simulink model "tongbukongzhi2"  (R2014b)
settings: Solver=ode45  StartTime=0.0  StopTime=10.0  RelTol=1e-3
undefined symbols (not defined in the file): sigbuilder_block
libraries: simulink x89, fuzblock x41
(part 5 of 5)

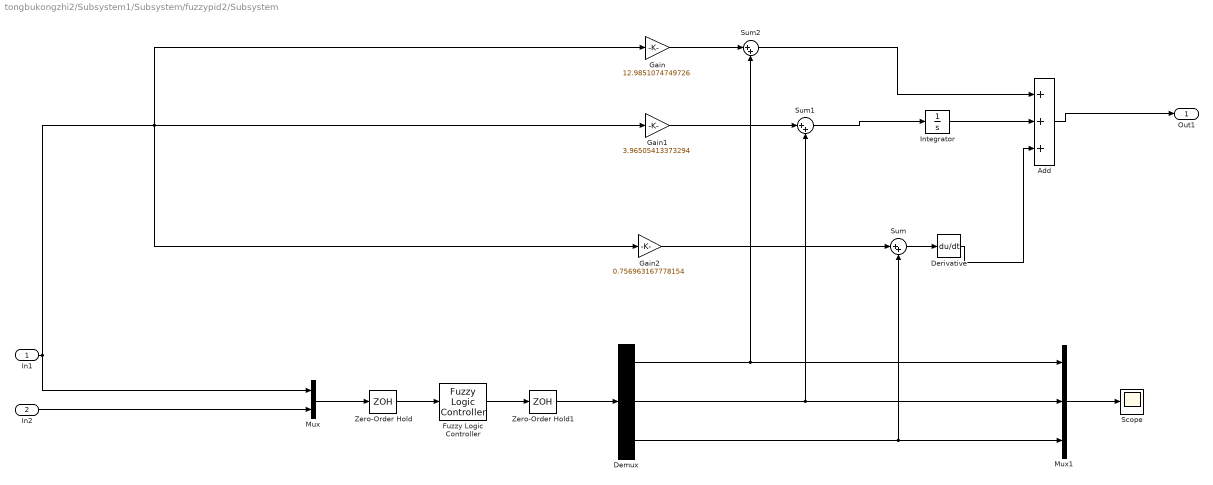
== system tongbukongzhi2/Subsystem1/Subsystem/fuzzypid2/Subsystem ==
  In1 : Inport
  In2 : Inport  Port=2
  Add : Sum  Inputs=+++
  Demux : Demux  Outputs=3
  Derivative : Derivative
  Fuzzy Logic Controller : fuzblock/Fuzzy Logic  Controller  fis=fuzzy1
  Gain : Gain  Gain=12.9851074749726
  Gain1 : Gain  Gain=3.96505413373294
  Gain2 : Gain  Gain=0.756963167778154
  Integrator : Integrator
  Mux : Mux  Inputs=2
  Mux1 : Mux  Inputs=3
  Scope : Scope
      settings: YMin=-0.2  YMax=0.05
  Sum : Sum  Inputs=|++
  Sum1 : Sum  Inputs=|++
  Sum2 : Sum  Inputs=|++
  Zero-Order Hold : ZeroOrderHold  SampleTime=0.1
  Zero-Order Hold1 : ZeroOrderHold  SampleTime=0.1
  Out1 : Outport
  wires:
  In1/1 -> Gain/1, Gain2/1, Gain1/1, Mux/1
  Derivative/1 -> Add/3
  Integrator/1 -> Add/2
  Add/1 -> Out1/1
  In2/1 -> Mux/2
  Gain/1 -> Sum2/1
  Sum2/1 -> Add/1
  Gain1/1 -> Sum1/1
  Sum1/1 -> Integrator/1
  Gain2/1 -> Sum/1
  Sum/1 -> Derivative/1
  Mux/1 -> Zero-Order Hold/1
  Fuzzy Logic Controller/1 -> Zero-Order Hold1/1
  Zero-Order Hold/1 -> Fuzzy Logic Controller/1
  Zero-Order Hold1/1 -> Demux/1
  Mux1/1 -> Scope/1
  Demux/3 -> Sum/2, Mux1/3
  Demux/2 -> Sum1/2, Mux1/2
  Demux/1 -> Mux1/1, Sum2/2

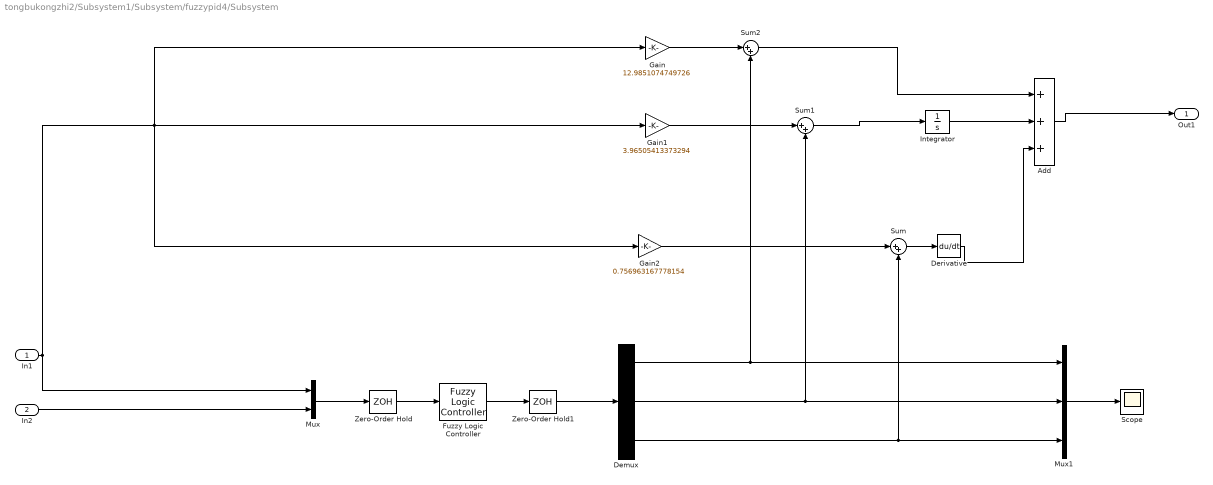
== system tongbukongzhi2/Subsystem1/Subsystem/fuzzypid4/Subsystem ==
  In1 : Inport
  In2 : Inport  Port=2
  Add : Sum  Inputs=+++
  Demux : Demux  Outputs=3
  Derivative : Derivative
  Fuzzy Logic Controller : fuzblock/Fuzzy Logic  Controller  fis=fuzzy1
  Gain : Gain  Gain=12.9851074749726
  Gain1 : Gain  Gain=3.96505413373294
  Gain2 : Gain  Gain=0.756963167778154
  Integrator : Integrator
  Mux : Mux  Inputs=2
  Mux1 : Mux  Inputs=3
  Scope : Scope
      settings: YMin=-0.2  YMax=0.05
  Sum : Sum  Inputs=|++
  Sum1 : Sum  Inputs=|++
  Sum2 : Sum  Inputs=|++
  Zero-Order Hold : ZeroOrderHold  SampleTime=0.1
  Zero-Order Hold1 : ZeroOrderHold  SampleTime=0.1
  Out1 : Outport
  wires:
  In1/1 -> Gain/1, Gain2/1, Gain1/1, Mux/1
  Derivative/1 -> Add/3
  Integrator/1 -> Add/2
  Add/1 -> Out1/1
  In2/1 -> Mux/2
  Gain/1 -> Sum2/1
  Sum2/1 -> Add/1
  Gain1/1 -> Sum1/1
  Sum1/1 -> Integrator/1
  Gain2/1 -> Sum/1
  Sum/1 -> Derivative/1
  Mux/1 -> Zero-Order Hold/1
  Fuzzy Logic Controller/1 -> Zero-Order Hold1/1
  Zero-Order Hold/1 -> Fuzzy Logic Controller/1
  Zero-Order Hold1/1 -> Demux/1
  Mux1/1 -> Scope/1
  Demux/3 -> Sum/2, Mux1/3
  Demux/2 -> Sum1/2, Mux1/2
  Demux/1 -> Mux1/1, Sum2/2

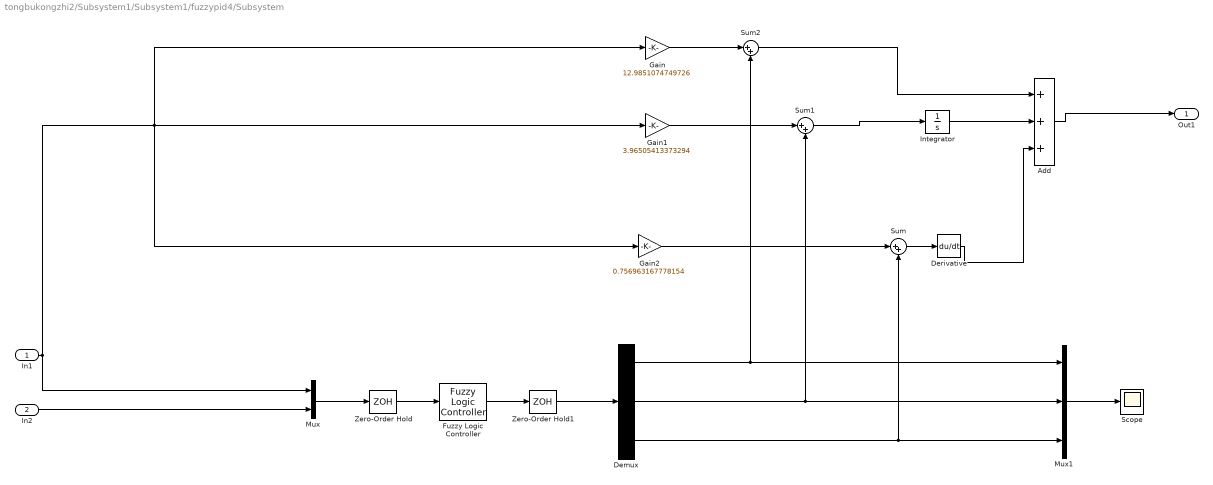
== system tongbukongzhi2/Subsystem1/Subsystem1/fuzzypid4/Subsystem ==
  In1 : Inport
  In2 : Inport  Port=2
  Add : Sum  Inputs=+++
  Demux : Demux  Outputs=3
  Derivative : Derivative
  Fuzzy Logic Controller : fuzblock/Fuzzy Logic  Controller  fis=fuzzy1
  Gain : Gain  Gain=12.9851074749726
  Gain1 : Gain  Gain=3.96505413373294
  Gain2 : Gain  Gain=0.756963167778154
  Integrator : Integrator
  Mux : Mux  Inputs=2
  Mux1 : Mux  Inputs=3
  Scope : Scope
      settings: YMin=-0.2  YMax=0.05
  Sum : Sum  Inputs=|++
  Sum1 : Sum  Inputs=|++
  Sum2 : Sum  Inputs=|++
  Zero-Order Hold : ZeroOrderHold  SampleTime=0.1
  Zero-Order Hold1 : ZeroOrderHold  SampleTime=0.1
  Out1 : Outport
  wires:
  In1/1 -> Gain/1, Gain2/1, Gain1/1, Mux/1
  Derivative/1 -> Add/3
  Integrator/1 -> Add/2
  Add/1 -> Out1/1
  In2/1 -> Mux/2
  Gain/1 -> Sum2/1
  Sum2/1 -> Add/1
  Gain1/1 -> Sum1/1
  Sum1/1 -> Integrator/1
  Gain2/1 -> Sum/1
  Sum/1 -> Derivative/1
  Mux/1 -> Zero-Order Hold/1
  Fuzzy Logic Controller/1 -> Zero-Order Hold1/1
  Zero-Order Hold/1 -> Fuzzy Logic Controller/1
  Zero-Order Hold1/1 -> Demux/1
  Mux1/1 -> Scope/1
  Demux/3 -> Sum/2, Mux1/3
  Demux/2 -> Sum1/2, Mux1/2
  Demux/1 -> Mux1/1, Sum2/2

== system tongbukongzhi2/Subsystem1/Subsystem1/fuzzypid5/Subsystem ==
  In1 : Inport
  In2 : Inport  Port=2
  Add : Sum  Inputs=+++
  Demux : Demux  Outputs=3
  Derivative : Derivative
  Fuzzy Logic Controller : fuzblock/Fuzzy Logic  Controller  fis=fuzzy1
  Gain : Gain  Gain=12.9851074749726
  Gain1 : Gain  Gain=3.96505413373294
  Gain2 : Gain  Gain=0.756963167778154
  Integrator : Integrator
  Mux : Mux  Inputs=2
  Mux1 : Mux  Inputs=3
  Scope : Scope
      settings: YMin=-0.2  YMax=0.05
  Sum : Sum  Inputs=|++
  Sum1 : Sum  Inputs=|++
  Sum2 : Sum  Inputs=|++
  Zero-Order Hold : ZeroOrderHold  SampleTime=0.1
  Zero-Order Hold1 : ZeroOrderHold  SampleTime=0.1
  Out1 : Outport
  wires:
  In1/1 -> Gain/1, Gain2/1, Gain1/1, Mux/1
  Derivative/1 -> Add/3
  Integrator/1 -> Add/2
  Add/1 -> Out1/1
  In2/1 -> Mux/2
  Gain/1 -> Sum2/1
  Sum2/1 -> Add/1
  Gain1/1 -> Sum1/1
  Sum1/1 -> Integrator/1
  Gain2/1 -> Sum/1
  Sum/1 -> Derivative/1
  Mux/1 -> Zero-Order Hold/1
  Fuzzy Logic Controller/1 -> Zero-Order Hold1/1
  Zero-Order Hold/1 -> Fuzzy Logic Controller/1
  Zero-Order Hold1/1 -> Demux/1
  Mux1/1 -> Scope/1
  Demux/3 -> Sum/2, Mux1/3
  Demux/2 -> Sum1/2, Mux1/2
  Demux/1 -> Mux1/1, Sum2/2

== system tongbukongzhi2/Subsystem1/Subsystem1/fuzzypid6/Subsystem ==
  In1 : Inport
  In2 : Inport  Port=2
  Add : Sum  Inputs=+++
  Demux : Demux  Outputs=3
  Derivative : Derivative
  Fuzzy Logic Controller : fuzblock/Fuzzy Logic  Controller  fis=fuzzy1
  Gain : Gain  Gain=12.9851074749726
  Gain1 : Gain  Gain=3.96505413373294
  Gain2 : Gain  Gain=0.756963167778154
  Integrator : Integrator
  Mux : Mux  Inputs=2
  Mux1 : Mux  Inputs=3
  Scope : Scope
      settings: YMin=-0.2  YMax=0.05
  Sum : Sum  Inputs=|++
  Sum1 : Sum  Inputs=|++
  Sum2 : Sum  Inputs=|++
  Zero-Order Hold : ZeroOrderHold  SampleTime=0.1
  Zero-Order Hold1 : ZeroOrderHold  SampleTime=0.1
  Out1 : Outport
  wires:
  In1/1 -> Gain/1, Gain2/1, Gain1/1, Mux/1
  Derivative/1 -> Add/3
  Integrator/1 -> Add/2
  Add/1 -> Out1/1
  In2/1 -> Mux/2
  Gain/1 -> Sum2/1
  Sum2/1 -> Add/1
  Gain1/1 -> Sum1/1
  Sum1/1 -> Integrator/1
  Gain2/1 -> Sum/1
  Sum/1 -> Derivative/1
  Mux/1 -> Zero-Order Hold/1
  Fuzzy Logic Controller/1 -> Zero-Order Hold1/1
  Zero-Order Hold/1 -> Fuzzy Logic Controller/1
  Zero-Order Hold1/1 -> Demux/1
  Mux1/1 -> Scope/1
  Demux/3 -> Sum/2, Mux1/3
  Demux/2 -> Sum1/2, Mux1/2
  Demux/1 -> Mux1/1, Sum2/2

== system tongbukongzhi2/Subsystem1/Subsystem12/fuzzypid1/Subsystem ==
  In1 : Inport
  In2 : Inport  Port=2
  Add : Sum  Inputs=+++
  Demux : Demux  Outputs=3
  Derivative : Derivative
  Fuzzy Logic Controller : fuzblock/Fuzzy Logic  Controller  fis=fuzzy1
  Gain : Gain  Gain=0.341898282831464
  Gain1 : Gain  Gain=4.22711463410027
  Gain2 : Gain  Gain=-0.0039506922991482
  Integrator : Integrator
  Mux : Mux  Inputs=2
  Mux1 : Mux  Inputs=3
  Scope : Scope
      settings: YMin=-0.2  YMax=0.05
  Sum : Sum  Inputs=|++
  Sum1 : Sum  Inputs=|++
  Sum2 : Sum  Inputs=|++
  Zero-Order Hold : ZeroOrderHold  SampleTime=0.1
  Zero-Order Hold1 : ZeroOrderHold  SampleTime=0.1
  Out1 : Outport
  wires:
  In1/1 -> Gain/1, Gain2/1, Gain1/1, Mux/1
  Derivative/1 -> Add/3
  Integrator/1 -> Add/2
  Add/1 -> Out1/1
  In2/1 -> Mux/2
  Gain/1 -> Sum2/1
  Sum2/1 -> Add/1
  Gain1/1 -> Sum1/1
  Sum1/1 -> Integrator/1
  Gain2/1 -> Sum/1
  Sum/1 -> Derivative/1
  Mux/1 -> Zero-Order Hold/1
  Fuzzy Logic Controller/1 -> Zero-Order Hold1/1
  Zero-Order Hold/1 -> Fuzzy Logic Controller/1
  Zero-Order Hold1/1 -> Demux/1
  Mux1/1 -> Scope/1
  Demux/3 -> Sum/2, Mux1/3
  Demux/2 -> Sum1/2, Mux1/2
  Demux/1 -> Mux1/1, Sum2/2

== system tongbukongzhi2/Subsystem1/Subsystem12/fuzzypid2/Subsystem ==
  In1 : Inport
  In2 : Inport  Port=2
  Add : Sum  Inputs=+++
  Demux : Demux  Outputs=3
  Derivative : Derivative
  Fuzzy Logic Controller : fuzblock/Fuzzy Logic  Controller  fis=fuzzy1
  Gain : Gain  Gain=0.341898282831464
  Gain1 : Gain  Gain=4.22711463410027
  Gain2 : Gain  Gain=-0.0039506922991482
  Integrator : Integrator
  Mux : Mux  Inputs=2
  Mux1 : Mux  Inputs=3
  Scope : Scope
      settings: YMin=-0.2  YMax=0.05
  Sum : Sum  Inputs=|++
  Sum1 : Sum  Inputs=|++
  Sum2 : Sum  Inputs=|++
  Zero-Order Hold : ZeroOrderHold  SampleTime=0.1
  Zero-Order Hold1 : ZeroOrderHold  SampleTime=0.1
  Out1 : Outport
  wires:
  In1/1 -> Gain/1, Gain2/1, Gain1/1, Mux/1
  Derivative/1 -> Add/3
  Integrator/1 -> Add/2
  Add/1 -> Out1/1
  In2/1 -> Mux/2
  Gain/1 -> Sum2/1
  Sum2/1 -> Add/1
  Gain1/1 -> Sum1/1
  Sum1/1 -> Integrator/1
  Gain2/1 -> Sum/1
  Sum/1 -> Derivative/1
  Mux/1 -> Zero-Order Hold/1
  Fuzzy Logic Controller/1 -> Zero-Order Hold1/1
  Zero-Order Hold/1 -> Fuzzy Logic Controller/1
  Zero-Order Hold1/1 -> Demux/1
  Mux1/1 -> Scope/1
  Demux/3 -> Sum/2, Mux1/3
  Demux/2 -> Sum1/2, Mux1/2
  Demux/1 -> Mux1/1, Sum2/2

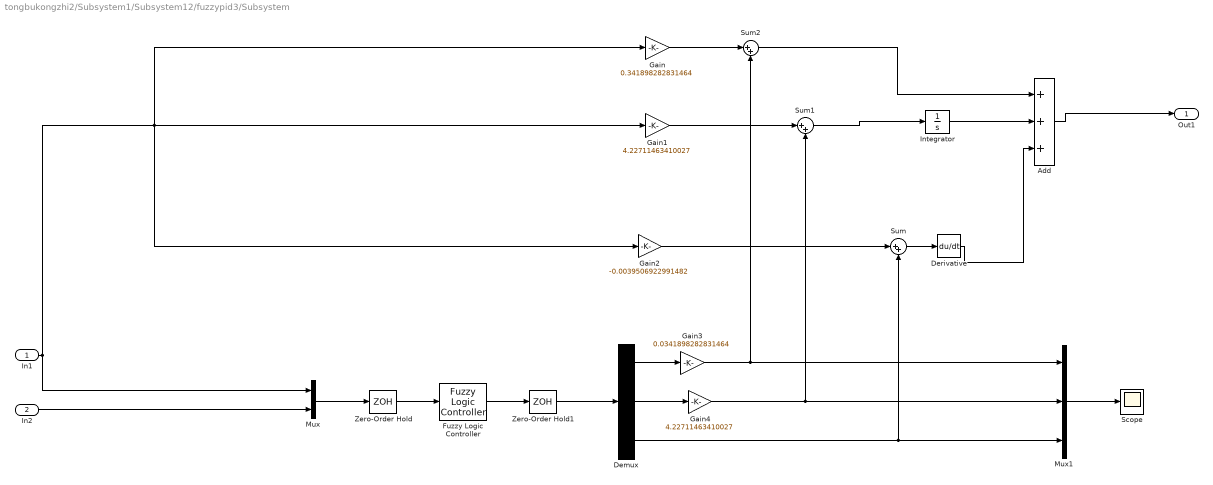
== system tongbukongzhi2/Subsystem1/Subsystem12/fuzzypid3/Subsystem ==
  In1 : Inport
  In2 : Inport  Port=2
  Add : Sum  Inputs=+++
  Demux : Demux  Outputs=3
  Derivative : Derivative
  Fuzzy Logic Controller : fuzblock/Fuzzy Logic  Controller  fis=fuzzy1
  Gain : Gain  Gain=0.341898282831464
  Gain1 : Gain  Gain=4.22711463410027
  Gain2 : Gain  Gain=-0.0039506922991482
  Gain3 : Gain  Gain=0.0341898282831464
  Gain4 : Gain  Gain=4.22711463410027
  Integrator : Integrator
  Mux : Mux  Inputs=2
  Mux1 : Mux  Inputs=3
  Scope : Scope
      settings: YMin=-0.2  YMax=0.05
  Sum : Sum  Inputs=|++
  Sum1 : Sum  Inputs=|++
  Sum2 : Sum  Inputs=|++
  Zero-Order Hold : ZeroOrderHold  SampleTime=0.1
  Zero-Order Hold1 : ZeroOrderHold  SampleTime=0.1
  Out1 : Outport
  wires:
  In1/1 -> Gain/1, Gain2/1, Gain1/1, Mux/1
  Derivative/1 -> Add/3
  Integrator/1 -> Add/2
  Add/1 -> Out1/1
  In2/1 -> Mux/2
  Gain/1 -> Sum2/1
  Sum2/1 -> Add/1
  Gain1/1 -> Sum1/1
  Sum1/1 -> Integrator/1
  Gain2/1 -> Sum/1
  Sum/1 -> Derivative/1
  Mux/1 -> Zero-Order Hold/1
  Fuzzy Logic Controller/1 -> Zero-Order Hold1/1
  Zero-Order Hold/1 -> Fuzzy Logic Controller/1
  Zero-Order Hold1/1 -> Demux/1
  Mux1/1 -> Scope/1
  Demux/3 -> Sum/2, Mux1/3
  Demux/2 -> Gain4/1
  Demux/1 -> Gain3/1
  Gain3/1 -> Mux1/1, Sum2/2
  Gain4/1 -> Sum1/2, Mux1/2

== system tongbukongzhi2/Subsystem1/Subsystem13/fuzzypid1/Subsystem ==
  In1 : Inport
  In2 : Inport  Port=2
  Add : Sum  Inputs=+++
  Demux : Demux  Outputs=3
  Derivative : Derivative
  Fuzzy Logic Controller : fuzblock/Fuzzy Logic  Controller  fis=fuzzy1
  Gain : Gain  Gain=0.341898282831464
  Gain1 : Gain  Gain=4.22711463410027
  Gain2 : Gain  Gain=-0.0039506922991482
  Integrator : Integrator
  Mux : Mux  Inputs=2
  Mux1 : Mux  Inputs=3
  Scope : Scope
      settings: YMin=-0.2  YMax=0.05
  Sum : Sum  Inputs=|++
  Sum1 : Sum  Inputs=|++
  Sum2 : Sum  Inputs=|++
  Zero-Order Hold : ZeroOrderHold  SampleTime=0.1
  Zero-Order Hold1 : ZeroOrderHold  SampleTime=0.1
  Out1 : Outport
  wires:
  In1/1 -> Gain/1, Gain2/1, Gain1/1, Mux/1
  Derivative/1 -> Add/3
  Integrator/1 -> Add/2
  Add/1 -> Out1/1
  In2/1 -> Mux/2
  Gain/1 -> Sum2/1
  Sum2/1 -> Add/1
  Gain1/1 -> Sum1/1
  Sum1/1 -> Integrator/1
  Gain2/1 -> Sum/1
  Sum/1 -> Derivative/1
  Mux/1 -> Zero-Order Hold/1
  Fuzzy Logic Controller/1 -> Zero-Order Hold1/1
  Zero-Order Hold/1 -> Fuzzy Logic Controller/1
  Zero-Order Hold1/1 -> Demux/1
  Mux1/1 -> Scope/1
  Demux/3 -> Sum/2, Mux1/3
  Demux/2 -> Sum1/2, Mux1/2
  Demux/1 -> Mux1/1, Sum2/2

== system tongbukongzhi2/Subsystem1/Subsystem13/fuzzypid2/Subsystem ==
  In1 : Inport
  In2 : Inport  Port=2
  Add : Sum  Inputs=+++
  Demux : Demux  Outputs=3
  Derivative : Derivative
  Fuzzy Logic Controller : fuzblock/Fuzzy Logic  Controller  fis=fuzzy1
  Gain : Gain  Gain=0.341898282831464
  Gain1 : Gain  Gain=4.22711463410027
  Gain2 : Gain  Gain=-0.0039506922991482
  Integrator : Integrator
  Mux : Mux  Inputs=2
  Mux1 : Mux  Inputs=3
  Scope : Scope
      settings: YMin=-0.2  YMax=0.05
  Sum : Sum  Inputs=|++
  Sum1 : Sum  Inputs=|++
  Sum2 : Sum  Inputs=|++
  Zero-Order Hold : ZeroOrderHold  SampleTime=0.1
  Zero-Order Hold1 : ZeroOrderHold  SampleTime=0.1
  Out1 : Outport
  wires:
  In1/1 -> Gain/1, Gain2/1, Gain1/1, Mux/1
  Derivative/1 -> Add/3
  Integrator/1 -> Add/2
  Add/1 -> Out1/1
  In2/1 -> Mux/2
  Gain/1 -> Sum2/1
  Sum2/1 -> Add/1
  Gain1/1 -> Sum1/1
  Sum1/1 -> Integrator/1
  Gain2/1 -> Sum/1
  Sum/1 -> Derivative/1
  Mux/1 -> Zero-Order Hold/1
  Fuzzy Logic Controller/1 -> Zero-Order Hold1/1
  Zero-Order Hold/1 -> Fuzzy Logic Controller/1
  Zero-Order Hold1/1 -> Demux/1
  Mux1/1 -> Scope/1
  Demux/3 -> Sum/2, Mux1/3
  Demux/2 -> Sum1/2, Mux1/2
  Demux/1 -> Mux1/1, Sum2/2

== system tongbukongzhi2/Subsystem1/Subsystem13/fuzzypid3/Subsystem ==
  In1 : Inport
  In2 : Inport  Port=2
  Add : Sum  Inputs=+++
  Demux : Demux  Outputs=3
  Derivative : Derivative
  Fuzzy Logic Controller : fuzblock/Fuzzy Logic  Controller  fis=fuzzy1
  Gain : Gain  Gain=0.341898282831464
  Gain1 : Gain  Gain=4.22711463410027
  Gain2 : Gain  Gain=-0.0039506922991482
  Integrator : Integrator
  Mux : Mux  Inputs=2
  Mux1 : Mux  Inputs=3
  Scope : Scope
      settings: YMin=-0.2  YMax=0.05
  Sum : Sum  Inputs=|++
  Sum1 : Sum  Inputs=|++
  Sum2 : Sum  Inputs=|++
  Zero-Order Hold : ZeroOrderHold  SampleTime=0.1
  Zero-Order Hold1 : ZeroOrderHold  SampleTime=0.1
  Out1 : Outport
  wires:
  In1/1 -> Gain/1, Gain2/1, Gain1/1, Mux/1
  Derivative/1 -> Add/3
  Integrator/1 -> Add/2
  Add/1 -> Out1/1
  In2/1 -> Mux/2
  Gain/1 -> Sum2/1
  Sum2/1 -> Add/1
  Gain1/1 -> Sum1/1
  Sum1/1 -> Integrator/1
  Gain2/1 -> Sum/1
  Sum/1 -> Derivative/1
  Mux/1 -> Zero-Order Hold/1
  Fuzzy Logic Controller/1 -> Zero-Order Hold1/1
  Zero-Order Hold/1 -> Fuzzy Logic Controller/1
  Zero-Order Hold1/1 -> Demux/1
  Mux1/1 -> Scope/1
  Demux/3 -> Sum/2, Mux1/3
  Demux/2 -> Sum1/2, Mux1/2
  Demux/1 -> Mux1/1, Sum2/2

== system tongbukongzhi2/Subsystem1/Subsystem14/fuzzypid1/Subsystem ==
  In1 : Inport
  In2 : Inport  Port=2
  Add : Sum  Inputs=+++
  Demux : Demux  Outputs=3
  Derivative : Derivative
  Fuzzy Logic Controller : fuzblock/Fuzzy Logic  Controller  fis=fuzzy1
  Gain : Gain  Gain=0.341898282831464
  Gain1 : Gain  Gain=4.22711463410027
  Gain2 : Gain  Gain=-0.0039506922991482
  Integrator : Integrator
  Mux : Mux  Inputs=2
  Mux1 : Mux  Inputs=3
  Scope : Scope
      settings: YMin=-0.2  YMax=0.05
  Sum : Sum  Inputs=|++
  Sum1 : Sum  Inputs=|++
  Sum2 : Sum  Inputs=|++
  Zero-Order Hold : ZeroOrderHold  SampleTime=0.1
  Zero-Order Hold1 : ZeroOrderHold  SampleTime=0.1
  Out1 : Outport
  wires:
  In1/1 -> Gain/1, Gain2/1, Gain1/1, Mux/1
  Derivative/1 -> Add/3
  Integrator/1 -> Add/2
  Add/1 -> Out1/1
  In2/1 -> Mux/2
  Gain/1 -> Sum2/1
  Sum2/1 -> Add/1
  Gain1/1 -> Sum1/1
  Sum1/1 -> Integrator/1
  Gain2/1 -> Sum/1
  Sum/1 -> Derivative/1
  Mux/1 -> Zero-Order Hold/1
  Fuzzy Logic Controller/1 -> Zero-Order Hold1/1
  Zero-Order Hold/1 -> Fuzzy Logic Controller/1
  Zero-Order Hold1/1 -> Demux/1
  Mux1/1 -> Scope/1
  Demux/3 -> Sum/2, Mux1/3
  Demux/2 -> Sum1/2, Mux1/2
  Demux/1 -> Mux1/1, Sum2/2

== system tongbukongzhi2/Subsystem1/Subsystem14/fuzzypid2/Subsystem ==
  In1 : Inport
  In2 : Inport  Port=2
  Add : Sum  Inputs=+++
  Demux : Demux  Outputs=3
  Derivative : Derivative
  Fuzzy Logic Controller : fuzblock/Fuzzy Logic  Controller  fis=fuzzy1
  Gain : Gain  Gain=0.341898282831464
  Gain1 : Gain  Gain=4.22711463410027
  Gain2 : Gain  Gain=-0.0039506922991482
  Integrator : Integrator
  Mux : Mux  Inputs=2
  Mux1 : Mux  Inputs=3
  Scope : Scope
      settings: YMin=-0.2  YMax=0.05
  Sum : Sum  Inputs=|++
  Sum1 : Sum  Inputs=|++
  Sum2 : Sum  Inputs=|++
  Zero-Order Hold : ZeroOrderHold  SampleTime=0.1
  Zero-Order Hold1 : ZeroOrderHold  SampleTime=0.1
  Out1 : Outport
  wires:
  In1/1 -> Gain/1, Gain2/1, Gain1/1, Mux/1
  Derivative/1 -> Add/3
  Integrator/1 -> Add/2
  Add/1 -> Out1/1
  In2/1 -> Mux/2
  Gain/1 -> Sum2/1
  Sum2/1 -> Add/1
  Gain1/1 -> Sum1/1
  Sum1/1 -> Integrator/1
  Gain2/1 -> Sum/1
  Sum/1 -> Derivative/1
  Mux/1 -> Zero-Order Hold/1
  Fuzzy Logic Controller/1 -> Zero-Order Hold1/1
  Zero-Order Hold/1 -> Fuzzy Logic Controller/1
  Zero-Order Hold1/1 -> Demux/1
  Mux1/1 -> Scope/1
  Demux/3 -> Sum/2, Mux1/3
  Demux/2 -> Sum1/2, Mux1/2
  Demux/1 -> Mux1/1, Sum2/2

== system tongbukongzhi2/Subsystem1/Subsystem14/fuzzypid3/Subsystem ==
  In1 : Inport
  In2 : Inport  Port=2
  Add : Sum  Inputs=+++
  Demux : Demux  Outputs=3
  Derivative : Derivative
  Fuzzy Logic Controller : fuzblock/Fuzzy Logic  Controller  fis=fuzzy1
  Gain : Gain  Gain=0.341898282831464
  Gain1 : Gain  Gain=4.22711463410027
  Gain2 : Gain  Gain=-0.0039506922991482
  Integrator : Integrator
  Mux : Mux  Inputs=2
  Mux1 : Mux  Inputs=3
  Scope : Scope
      settings: YMin=-0.2  YMax=0.05
  Sum : Sum  Inputs=|++
  Sum1 : Sum  Inputs=|++
  Sum2 : Sum  Inputs=|++
  Zero-Order Hold : ZeroOrderHold  SampleTime=0.1
  Zero-Order Hold1 : ZeroOrderHold  SampleTime=0.1
  Out1 : Outport
  wires:
  In1/1 -> Gain/1, Gain2/1, Gain1/1, Mux/1
  Derivative/1 -> Add/3
  Integrator/1 -> Add/2
  Add/1 -> Out1/1
  In2/1 -> Mux/2
  Gain/1 -> Sum2/1
  Sum2/1 -> Add/1
  Gain1/1 -> Sum1/1
  Sum1/1 -> Integrator/1
  Gain2/1 -> Sum/1
  Sum/1 -> Derivative/1
  Mux/1 -> Zero-Order Hold/1
  Fuzzy Logic Controller/1 -> Zero-Order Hold1/1
  Zero-Order Hold/1 -> Fuzzy Logic Controller/1
  Zero-Order Hold1/1 -> Demux/1
  Mux1/1 -> Scope/1
  Demux/3 -> Sum/2, Mux1/3
  Demux/2 -> Sum1/2, Mux1/2
  Demux/1 -> Mux1/1, Sum2/2

== system tongbukongzhi2/Subsystem1/Subsystem15/fuzzypid1/Subsystem ==
  In1 : Inport
  In2 : Inport  Port=2
  Add : Sum  Inputs=+++
  Demux : Demux  Outputs=3
  Derivative : Derivative
  Fuzzy Logic Controller : fuzblock/Fuzzy Logic  Controller  fis=fuzzy1
  Gain : Gain  Gain=0.341898282831464
  Gain1 : Gain  Gain=4.22711463410027
  Gain2 : Gain  Gain=-0.0039506922991482
  Integrator : Integrator
  Mux : Mux  Inputs=2
  Mux1 : Mux  Inputs=3
  Scope : Scope
      settings: YMin=-0.2  YMax=0.05
  Sum : Sum  Inputs=|++
  Sum1 : Sum  Inputs=|++
  Sum2 : Sum  Inputs=|++
  Zero-Order Hold : ZeroOrderHold  SampleTime=0.1
  Zero-Order Hold1 : ZeroOrderHold  SampleTime=0.1
  Out1 : Outport
  wires:
  In1/1 -> Gain/1, Gain2/1, Gain1/1, Mux/1
  Derivative/1 -> Add/3
  Integrator/1 -> Add/2
  Add/1 -> Out1/1
  In2/1 -> Mux/2
  Gain/1 -> Sum2/1
  Sum2/1 -> Add/1
  Gain1/1 -> Sum1/1
  Sum1/1 -> Integrator/1
  Gain2/1 -> Sum/1
  Sum/1 -> Derivative/1
  Mux/1 -> Zero-Order Hold/1
  Fuzzy Logic Controller/1 -> Zero-Order Hold1/1
  Zero-Order Hold/1 -> Fuzzy Logic Controller/1
  Zero-Order Hold1/1 -> Demux/1
  Mux1/1 -> Scope/1
  Demux/3 -> Sum/2, Mux1/3
  Demux/2 -> Sum1/2, Mux1/2
  Demux/1 -> Mux1/1, Sum2/2

== system tongbukongzhi2/Subsystem1/Subsystem15/fuzzypid2/Subsystem ==
  In1 : Inport
  In2 : Inport  Port=2
  Add : Sum  Inputs=+++
  Demux : Demux  Outputs=3
  Derivative : Derivative
  Fuzzy Logic Controller : fuzblock/Fuzzy Logic  Controller  fis=fuzzy1
  Gain : Gain  Gain=0.341898282831464
  Gain1 : Gain  Gain=4.22711463410027
  Gain2 : Gain  Gain=-0.0039506922991482
  Integrator : Integrator
  Mux : Mux  Inputs=2
  Mux1 : Mux  Inputs=3
  Scope : Scope
      settings: YMin=-0.2  YMax=0.05
  Sum : Sum  Inputs=|++
  Sum1 : Sum  Inputs=|++
  Sum2 : Sum  Inputs=|++
  Zero-Order Hold : ZeroOrderHold  SampleTime=0.1
  Zero-Order Hold1 : ZeroOrderHold  SampleTime=0.1
  Out1 : Outport
  wires:
  In1/1 -> Gain/1, Gain2/1, Gain1/1, Mux/1
  Derivative/1 -> Add/3
  Integrator/1 -> Add/2
  Add/1 -> Out1/1
  In2/1 -> Mux/2
  Gain/1 -> Sum2/1
  Sum2/1 -> Add/1
  Gain1/1 -> Sum1/1
  Sum1/1 -> Integrator/1
  Gain2/1 -> Sum/1
  Sum/1 -> Derivative/1
  Mux/1 -> Zero-Order Hold/1
  Fuzzy Logic Controller/1 -> Zero-Order Hold1/1
  Zero-Order Hold/1 -> Fuzzy Logic Controller/1
  Zero-Order Hold1/1 -> Demux/1
  Mux1/1 -> Scope/1
  Demux/3 -> Sum/2, Mux1/3
  Demux/2 -> Sum1/2, Mux1/2
  Demux/1 -> Mux1/1, Sum2/2

== system tongbukongzhi2/Subsystem1/Subsystem15/fuzzypid3/Subsystem ==
  In1 : Inport
  In2 : Inport  Port=2
  Add : Sum  Inputs=+++
  Demux : Demux  Outputs=3
  Derivative : Derivative
  Fuzzy Logic Controller : fuzblock/Fuzzy Logic  Controller  fis=fuzzy1
  Gain : Gain  Gain=0.341898282831464
  Gain1 : Gain  Gain=4.22711463410027
  Gain2 : Gain  Gain=-0.0039506922991482
  Integrator : Integrator
  Mux : Mux  Inputs=2
  Mux1 : Mux  Inputs=3
  Scope : Scope
      settings: YMin=-0.2  YMax=0.05
  Sum : Sum  Inputs=|++
  Sum1 : Sum  Inputs=|++
  Sum2 : Sum  Inputs=|++
  Zero-Order Hold : ZeroOrderHold  SampleTime=0.1
  Zero-Order Hold1 : ZeroOrderHold  SampleTime=0.1
  Out1 : Outport
  wires:
  In1/1 -> Gain/1, Gain2/1, Gain1/1, Mux/1
  Derivative/1 -> Add/3
  Integrator/1 -> Add/2
  Add/1 -> Out1/1
  In2/1 -> Mux/2
  Gain/1 -> Sum2/1
  Sum2/1 -> Add/1
  Gain1/1 -> Sum1/1
  Sum1/1 -> Integrator/1
  Gain2/1 -> Sum/1
  Sum/1 -> Derivative/1
  Mux/1 -> Zero-Order Hold/1
  Fuzzy Logic Controller/1 -> Zero-Order Hold1/1
  Zero-Order Hold/1 -> Fuzzy Logic Controller/1
  Zero-Order Hold1/1 -> Demux/1
  Mux1/1 -> Scope/1
  Demux/3 -> Sum/2, Mux1/3
  Demux/2 -> Sum1/2, Mux1/2
  Demux/1 -> Mux1/1, Sum2/2

== system tongbukongzhi2/Subsystem1/Subsystem16/fuzzypid1/Subsystem ==
  In1 : Inport
  In2 : Inport  Port=2
  Add : Sum  Inputs=+++
  Demux : Demux  Outputs=3
  Derivative : Derivative
  Fuzzy Logic Controller : fuzblock/Fuzzy Logic  Controller  fis=fuzzy1
  Gain : Gain  Gain=12.9851074749726
  Gain1 : Gain  Gain=3.96505413373294
  Gain2 : Gain  Gain=0.756963167778154
  Integrator : Integrator
  Mux : Mux  Inputs=2
  Mux1 : Mux  Inputs=3
  Scope : Scope
      settings: YMin=-0.2  YMax=0.05
  Sum : Sum  Inputs=|++
  Sum1 : Sum  Inputs=|++
  Sum2 : Sum  Inputs=|++
  Zero-Order Hold : ZeroOrderHold  SampleTime=0.1
  Zero-Order Hold1 : ZeroOrderHold  SampleTime=0.1
  Out1 : Outport
  wires:
  In1/1 -> Gain/1, Gain2/1, Gain1/1, Mux/1
  Derivative/1 -> Add/3
  Integrator/1 -> Add/2
  Add/1 -> Out1/1
  In2/1 -> Mux/2
  Gain/1 -> Sum2/1
  Sum2/1 -> Add/1
  Gain1/1 -> Sum1/1
  Sum1/1 -> Integrator/1
  Gain2/1 -> Sum/1
  Sum/1 -> Derivative/1
  Mux/1 -> Zero-Order Hold/1
  Fuzzy Logic Controller/1 -> Zero-Order Hold1/1
  Zero-Order Hold/1 -> Fuzzy Logic Controller/1
  Zero-Order Hold1/1 -> Demux/1
  Mux1/1 -> Scope/1
  Demux/3 -> Sum/2, Mux1/3
  Demux/2 -> Sum1/2, Mux1/2
  Demux/1 -> Mux1/1, Sum2/2

== system tongbukongzhi2/Subsystem1/Subsystem16/fuzzypid2/Subsystem ==
  In1 : Inport
  In2 : Inport  Port=2
  Add : Sum  Inputs=+++
  Demux : Demux  Outputs=3
  Derivative : Derivative
  Fuzzy Logic Controller : fuzblock/Fuzzy Logic  Controller  fis=fuzzy1
  Gain : Gain  Gain=12.9851074749726
  Gain1 : Gain  Gain=3.96505413373294
  Gain2 : Gain  Gain=0.756963167778154
  Integrator : Integrator
  Mux : Mux  Inputs=2
  Mux1 : Mux  Inputs=3
  Scope : Scope
      settings: YMin=-0.2  YMax=0.05
  Sum : Sum  Inputs=|++
  Sum1 : Sum  Inputs=|++
  Sum2 : Sum  Inputs=|++
  Zero-Order Hold : ZeroOrderHold  SampleTime=0.1
  Zero-Order Hold1 : ZeroOrderHold  SampleTime=0.1
  Out1 : Outport
  wires:
  In1/1 -> Gain/1, Gain2/1, Gain1/1, Mux/1
  Derivative/1 -> Add/3
  Integrator/1 -> Add/2
  Add/1 -> Out1/1
  In2/1 -> Mux/2
  Gain/1 -> Sum2/1
  Sum2/1 -> Add/1
  Gain1/1 -> Sum1/1
  Sum1/1 -> Integrator/1
  Gain2/1 -> Sum/1
  Sum/1 -> Derivative/1
  Mux/1 -> Zero-Order Hold/1
  Fuzzy Logic Controller/1 -> Zero-Order Hold1/1
  Zero-Order Hold/1 -> Fuzzy Logic Controller/1
  Zero-Order Hold1/1 -> Demux/1
  Mux1/1 -> Scope/1
  Demux/3 -> Sum/2, Mux1/3
  Demux/2 -> Sum1/2, Mux1/2
  Demux/1 -> Mux1/1, Sum2/2

== system tongbukongzhi2/Subsystem1/Subsystem16/fuzzypid4/Subsystem ==
  In1 : Inport
  In2 : Inport  Port=2
  Add : Sum  Inputs=+++
  Demux : Demux  Outputs=3
  Derivative : Derivative
  Fuzzy Logic Controller : fuzblock/Fuzzy Logic  Controller  fis=fuzzy1
  Gain : Gain  Gain=12.9851074749726
  Gain1 : Gain  Gain=3.96505413373294
  Gain2 : Gain  Gain=0.756963167778154
  Integrator : Integrator
  Mux : Mux  Inputs=2
  Mux1 : Mux  Inputs=3
  Scope : Scope
      settings: YMin=-0.2  YMax=0.05
  Sum : Sum  Inputs=|++
  Sum1 : Sum  Inputs=|++
  Sum2 : Sum  Inputs=|++
  Zero-Order Hold : ZeroOrderHold  SampleTime=0.1
  Zero-Order Hold1 : ZeroOrderHold  SampleTime=0.1
  Out1 : Outport
  wires:
  In1/1 -> Gain/1, Gain2/1, Gain1/1, Mux/1
  Derivative/1 -> Add/3
  Integrator/1 -> Add/2
  Add/1 -> Out1/1
  In2/1 -> Mux/2
  Gain/1 -> Sum2/1
  Sum2/1 -> Add/1
  Gain1/1 -> Sum1/1
  Sum1/1 -> Integrator/1
  Gain2/1 -> Sum/1
  Sum/1 -> Derivative/1
  Mux/1 -> Zero-Order Hold/1
  Fuzzy Logic Controller/1 -> Zero-Order Hold1/1
  Zero-Order Hold/1 -> Fuzzy Logic Controller/1
  Zero-Order Hold1/1 -> Demux/1
  Mux1/1 -> Scope/1
  Demux/3 -> Sum/2, Mux1/3
  Demux/2 -> Sum1/2, Mux1/2
  Demux/1 -> Mux1/1, Sum2/2

== system tongbukongzhi2/Subsystem1/Subsystem17/fuzzypid4/Subsystem ==
  In1 : Inport
  In2 : Inport  Port=2
  Add : Sum  Inputs=+++
  Demux : Demux  Outputs=3
  Derivative : Derivative
  Fuzzy Logic Controller : fuzblock/Fuzzy Logic  Controller  fis=fuzzy1
  Gain : Gain  Gain=12.9851074749726
  Gain1 : Gain  Gain=3.96505413373294
  Gain2 : Gain  Gain=0.756963167778154
  Integrator : Integrator
  Mux : Mux  Inputs=2
  Mux1 : Mux  Inputs=3
  Scope : Scope
      settings: YMin=-0.2  YMax=0.05
  Sum : Sum  Inputs=|++
  Sum1 : Sum  Inputs=|++
  Sum2 : Sum  Inputs=|++
  Zero-Order Hold : ZeroOrderHold  SampleTime=0.1
  Zero-Order Hold1 : ZeroOrderHold  SampleTime=0.1
  Out1 : Outport
  wires:
  In1/1 -> Gain/1, Gain2/1, Gain1/1, Mux/1
  Derivative/1 -> Add/3
  Integrator/1 -> Add/2
  Add/1 -> Out1/1
  In2/1 -> Mux/2
  Gain/1 -> Sum2/1
  Sum2/1 -> Add/1
  Gain1/1 -> Sum1/1
  Sum1/1 -> Integrator/1
  Gain2/1 -> Sum/1
  Sum/1 -> Derivative/1
  Mux/1 -> Zero-Order Hold/1
  Fuzzy Logic Controller/1 -> Zero-Order Hold1/1
  Zero-Order Hold/1 -> Fuzzy Logic Controller/1
  Zero-Order Hold1/1 -> Demux/1
  Mux1/1 -> Scope/1
  Demux/3 -> Sum/2, Mux1/3
  Demux/2 -> Sum1/2, Mux1/2
  Demux/1 -> Mux1/1, Sum2/2

== system tongbukongzhi2/Subsystem1/Subsystem17/fuzzypid5/Subsystem ==
  In1 : Inport
  In2 : Inport  Port=2
  Add : Sum  Inputs=+++
  Demux : Demux  Outputs=3
  Derivative : Derivative
  Fuzzy Logic Controller : fuzblock/Fuzzy Logic  Controller  fis=fuzzy1
  Gain : Gain  Gain=12.9851074749726
  Gain1 : Gain  Gain=3.96505413373294
  Gain2 : Gain  Gain=0.756963167778154
  Integrator : Integrator
  Mux : Mux  Inputs=2
  Mux1 : Mux  Inputs=3
  Scope : Scope
      settings: YMin=-0.2  YMax=0.05
  Sum : Sum  Inputs=|++
  Sum1 : Sum  Inputs=|++
  Sum2 : Sum  Inputs=|++
  Zero-Order Hold : ZeroOrderHold  SampleTime=0.1
  Zero-Order Hold1 : ZeroOrderHold  SampleTime=0.1
  Out1 : Outport
  wires:
  In1/1 -> Gain/1, Gain2/1, Gain1/1, Mux/1
  Derivative/1 -> Add/3
  Integrator/1 -> Add/2
  Add/1 -> Out1/1
  In2/1 -> Mux/2
  Gain/1 -> Sum2/1
  Sum2/1 -> Add/1
  Gain1/1 -> Sum1/1
  Sum1/1 -> Integrator/1
  Gain2/1 -> Sum/1
  Sum/1 -> Derivative/1
  Mux/1 -> Zero-Order Hold/1
  Fuzzy Logic Controller/1 -> Zero-Order Hold1/1
  Zero-Order Hold/1 -> Fuzzy Logic Controller/1
  Zero-Order Hold1/1 -> Demux/1
  Mux1/1 -> Scope/1
  Demux/3 -> Sum/2, Mux1/3
  Demux/2 -> Sum1/2, Mux1/2
  Demux/1 -> Mux1/1, Sum2/2

== system tongbukongzhi2/Subsystem1/Subsystem17/fuzzypid6/Subsystem ==
  In1 : Inport
  In2 : Inport  Port=2
  Add : Sum  Inputs=+++
  Demux : Demux  Outputs=3
  Derivative : Derivative
  Fuzzy Logic Controller : fuzblock/Fuzzy Logic  Controller  fis=fuzzy1
  Gain : Gain  Gain=12.9851074749726
  Gain1 : Gain  Gain=3.96505413373294
  Gain2 : Gain  Gain=0.756963167778154
  Integrator : Integrator
  Mux : Mux  Inputs=2
  Mux1 : Mux  Inputs=3
  Scope : Scope
      settings: YMin=-0.2  YMax=0.05
  Sum : Sum  Inputs=|++
  Sum1 : Sum  Inputs=|++
  Sum2 : Sum  Inputs=|++
  Zero-Order Hold : ZeroOrderHold  SampleTime=0.1
  Zero-Order Hold1 : ZeroOrderHold  SampleTime=0.1
  Out1 : Outport
  wires:
  In1/1 -> Gain/1, Gain2/1, Gain1/1, Mux/1
  Derivative/1 -> Add/3
  Integrator/1 -> Add/2
  Add/1 -> Out1/1
  In2/1 -> Mux/2
  Gain/1 -> Sum2/1
  Sum2/1 -> Add/1
  Gain1/1 -> Sum1/1
  Sum1/1 -> Integrator/1
  Gain2/1 -> Sum/1
  Sum/1 -> Derivative/1
  Mux/1 -> Zero-Order Hold/1
  Fuzzy Logic Controller/1 -> Zero-Order Hold1/1
  Zero-Order Hold/1 -> Fuzzy Logic Controller/1
  Zero-Order Hold1/1 -> Demux/1
  Mux1/1 -> Scope/1
  Demux/3 -> Sum/2, Mux1/3
  Demux/2 -> Sum1/2, Mux1/2
  Demux/1 -> Mux1/1, Sum2/2

== system tongbukongzhi2/Subsystem1/Subsystem18/fuzzypid4/Subsystem ==
  In1 : Inport
  In2 : Inport  Port=2
  Add : Sum  Inputs=+++
  Demux : Demux  Outputs=3
  Derivative : Derivative
  Fuzzy Logic Controller : fuzblock/Fuzzy Logic  Controller  fis=fuzzy1
  Gain : Gain  Gain=12.9851074749726
  Gain1 : Gain  Gain=3.96505413373294
  Gain2 : Gain  Gain=0.756963167778154
  Integrator : Integrator
  Mux : Mux  Inputs=2
  Mux1 : Mux  Inputs=3
  Scope : Scope
      settings: YMin=-0.2  YMax=0.05
  Sum : Sum  Inputs=|++
  Sum1 : Sum  Inputs=|++
  Sum2 : Sum  Inputs=|++
  Zero-Order Hold : ZeroOrderHold  SampleTime=0.1
  Zero-Order Hold1 : ZeroOrderHold  SampleTime=0.1
  Out1 : Outport
  wires:
  In1/1 -> Gain/1, Gain2/1, Gain1/1, Mux/1
  Derivative/1 -> Add/3
  Integrator/1 -> Add/2
  Add/1 -> Out1/1
  In2/1 -> Mux/2
  Gain/1 -> Sum2/1
  Sum2/1 -> Add/1
  Gain1/1 -> Sum1/1
  Sum1/1 -> Integrator/1
  Gain2/1 -> Sum/1
  Sum/1 -> Derivative/1
  Mux/1 -> Zero-Order Hold/1
  Fuzzy Logic Controller/1 -> Zero-Order Hold1/1
  Zero-Order Hold/1 -> Fuzzy Logic Controller/1
  Zero-Order Hold1/1 -> Demux/1
  Mux1/1 -> Scope/1
  Demux/3 -> Sum/2, Mux1/3
  Demux/2 -> Sum1/2, Mux1/2
  Demux/1 -> Mux1/1, Sum2/2

== system tongbukongzhi2/Subsystem1/Subsystem18/fuzzypid5/Subsystem ==
  In1 : Inport
  In2 : Inport  Port=2
  Add : Sum  Inputs=+++
  Demux : Demux  Outputs=3
  Derivative : Derivative
  Fuzzy Logic Controller : fuzblock/Fuzzy Logic  Controller  fis=fuzzy1
  Gain : Gain  Gain=12.9851074749726
  Gain1 : Gain  Gain=3.96505413373294
  Gain2 : Gain  Gain=0.756963167778154
  Integrator : Integrator
  Mux : Mux  Inputs=2
  Mux1 : Mux  Inputs=3
  Scope : Scope
      settings: YMin=-0.2  YMax=0.05
  Sum : Sum  Inputs=|++
  Sum1 : Sum  Inputs=|++
  Sum2 : Sum  Inputs=|++
  Zero-Order Hold : ZeroOrderHold  SampleTime=0.1
  Zero-Order Hold1 : ZeroOrderHold  SampleTime=0.1
  Out1 : Outport
  wires:
  In1/1 -> Gain/1, Gain2/1, Gain1/1, Mux/1
  Derivative/1 -> Add/3
  Integrator/1 -> Add/2
  Add/1 -> Out1/1
  In2/1 -> Mux/2
  Gain/1 -> Sum2/1
  Sum2/1 -> Add/1
  Gain1/1 -> Sum1/1
  Sum1/1 -> Integrator/1
  Gain2/1 -> Sum/1
  Sum/1 -> Derivative/1
  Mux/1 -> Zero-Order Hold/1
  Fuzzy Logic Controller/1 -> Zero-Order Hold1/1
  Zero-Order Hold/1 -> Fuzzy Logic Controller/1
  Zero-Order Hold1/1 -> Demux/1
  Mux1/1 -> Scope/1
  Demux/3 -> Sum/2, Mux1/3
  Demux/2 -> Sum1/2, Mux1/2
  Demux/1 -> Mux1/1, Sum2/2

== system tongbukongzhi2/Subsystem1/Subsystem18/fuzzypid6/Subsystem ==
  In1 : Inport
  In2 : Inport  Port=2
  Add : Sum  Inputs=+++
  Demux : Demux  Outputs=3
  Derivative : Derivative
  Fuzzy Logic Controller : fuzblock/Fuzzy Logic  Controller  fis=fuzzy1
  Gain : Gain  Gain=12.9851074749726
  Gain1 : Gain  Gain=3.96505413373294
  Gain2 : Gain  Gain=0.756963167778154
  Integrator : Integrator
  Mux : Mux  Inputs=2
  Mux1 : Mux  Inputs=3
  Scope : Scope
      settings: YMin=-0.2  YMax=0.05
  Sum : Sum  Inputs=|++
  Sum1 : Sum  Inputs=|++
  Sum2 : Sum  Inputs=|++
  Zero-Order Hold : ZeroOrderHold  SampleTime=0.1
  Zero-Order Hold1 : ZeroOrderHold  SampleTime=0.1
  Out1 : Outport
  wires:
  In1/1 -> Gain/1, Gain2/1, Gain1/1, Mux/1
  Derivative/1 -> Add/3
  Integrator/1 -> Add/2
  Add/1 -> Out1/1
  In2/1 -> Mux/2
  Gain/1 -> Sum2/1
  Sum2/1 -> Add/1
  Gain1/1 -> Sum1/1
  Sum1/1 -> Integrator/1
  Gain2/1 -> Sum/1
  Sum/1 -> Derivative/1
  Mux/1 -> Zero-Order Hold/1
  Fuzzy Logic Controller/1 -> Zero-Order Hold1/1
  Zero-Order Hold/1 -> Fuzzy Logic Controller/1
  Zero-Order Hold1/1 -> Demux/1
  Mux1/1 -> Scope/1
  Demux/3 -> Sum/2, Mux1/3
  Demux/2 -> Sum1/2, Mux1/2
  Demux/1 -> Mux1/1, Sum2/2

== system tongbukongzhi2/Subsystem1/Subsystem19/fuzzypid4/Subsystem ==
  In1 : Inport
  In2 : Inport  Port=2
  Add : Sum  Inputs=+++
  Demux : Demux  Outputs=3
  Derivative : Derivative
  Fuzzy Logic Controller : fuzblock/Fuzzy Logic  Controller  fis=fuzzy1
  Gain : Gain  Gain=12.9851074749726
  Gain1 : Gain  Gain=3.96505413373294
  Gain2 : Gain  Gain=0.756963167778154
  Integrator : Integrator
  Mux : Mux  Inputs=2
  Mux1 : Mux  Inputs=3
  Scope : Scope
      settings: YMin=-0.2  YMax=0.05
  Sum : Sum  Inputs=|++
  Sum1 : Sum  Inputs=|++
  Sum2 : Sum  Inputs=|++
  Zero-Order Hold : ZeroOrderHold  SampleTime=0.1
  Zero-Order Hold1 : ZeroOrderHold  SampleTime=0.1
  Out1 : Outport
  wires:
  In1/1 -> Gain/1, Gain2/1, Gain1/1, Mux/1
  Derivative/1 -> Add/3
  Integrator/1 -> Add/2
  Add/1 -> Out1/1
  In2/1 -> Mux/2
  Gain/1 -> Sum2/1
  Sum2/1 -> Add/1
  Gain1/1 -> Sum1/1
  Sum1/1 -> Integrator/1
  Gain2/1 -> Sum/1
  Sum/1 -> Derivative/1
  Mux/1 -> Zero-Order Hold/1
  Fuzzy Logic Controller/1 -> Zero-Order Hold1/1
  Zero-Order Hold/1 -> Fuzzy Logic Controller/1
  Zero-Order Hold1/1 -> Demux/1
  Mux1/1 -> Scope/1
  Demux/3 -> Sum/2, Mux1/3
  Demux/2 -> Sum1/2, Mux1/2
  Demux/1 -> Mux1/1, Sum2/2

== system tongbukongzhi2/Subsystem1/Subsystem19/fuzzypid5/Subsystem ==
  In1 : Inport
  In2 : Inport  Port=2
  Add : Sum  Inputs=+++
  Demux : Demux  Outputs=3
  Derivative : Derivative
  Fuzzy Logic Controller : fuzblock/Fuzzy Logic  Controller  fis=fuzzy1
  Gain : Gain  Gain=12.9851074749726
  Gain1 : Gain  Gain=3.96505413373294
  Gain2 : Gain  Gain=0.756963167778154
  Integrator : Integrator
  Mux : Mux  Inputs=2
  Mux1 : Mux  Inputs=3
  Scope : Scope
      settings: YMin=-0.2  YMax=0.05
  Sum : Sum  Inputs=|++
  Sum1 : Sum  Inputs=|++
  Sum2 : Sum  Inputs=|++
  Zero-Order Hold : ZeroOrderHold  SampleTime=0.1
  Zero-Order Hold1 : ZeroOrderHold  SampleTime=0.1
  Out1 : Outport
  wires:
  In1/1 -> Gain/1, Gain2/1, Gain1/1, Mux/1
  Derivative/1 -> Add/3
  Integrator/1 -> Add/2
  Add/1 -> Out1/1
  In2/1 -> Mux/2
  Gain/1 -> Sum2/1
  Sum2/1 -> Add/1
  Gain1/1 -> Sum1/1
  Sum1/1 -> Integrator/1
  Gain2/1 -> Sum/1
  Sum/1 -> Derivative/1
  Mux/1 -> Zero-Order Hold/1
  Fuzzy Logic Controller/1 -> Zero-Order Hold1/1
  Zero-Order Hold/1 -> Fuzzy Logic Controller/1
  Zero-Order Hold1/1 -> Demux/1
  Mux1/1 -> Scope/1
  Demux/3 -> Sum/2, Mux1/3
  Demux/2 -> Sum1/2, Mux1/2
  Demux/1 -> Mux1/1, Sum2/2

== system tongbukongzhi2/Subsystem1/Subsystem19/fuzzypid6/Subsystem ==
  In1 : Inport
  In2 : Inport  Port=2
  Add : Sum  Inputs=+++
  Demux : Demux  Outputs=3
  Derivative : Derivative
  Fuzzy Logic Controller : fuzblock/Fuzzy Logic  Controller  fis=fuzzy1
  Gain : Gain  Gain=12.9851074749726
  Gain1 : Gain  Gain=3.96505413373294
  Gain2 : Gain  Gain=0.756963167778154
  Integrator : Integrator
  Mux : Mux  Inputs=2
  Mux1 : Mux  Inputs=3
  Scope : Scope
      settings: YMin=-0.2  YMax=0.05
  Sum : Sum  Inputs=|++
  Sum1 : Sum  Inputs=|++
  Sum2 : Sum  Inputs=|++
  Zero-Order Hold : ZeroOrderHold  SampleTime=0.1
  Zero-Order Hold1 : ZeroOrderHold  SampleTime=0.1
  Out1 : Outport
  wires:
  In1/1 -> Gain/1, Gain2/1, Gain1/1, Mux/1
  Derivative/1 -> Add/3
  Integrator/1 -> Add/2
  Add/1 -> Out1/1
  In2/1 -> Mux/2
  Gain/1 -> Sum2/1
  Sum2/1 -> Add/1
  Gain1/1 -> Sum1/1
  Sum1/1 -> Integrator/1
  Gain2/1 -> Sum/1
  Sum/1 -> Derivative/1
  Mux/1 -> Zero-Order Hold/1
  Fuzzy Logic Controller/1 -> Zero-Order Hold1/1
  Zero-Order Hold/1 -> Fuzzy Logic Controller/1
  Zero-Order Hold1/1 -> Demux/1
  Mux1/1 -> Scope/1
  Demux/3 -> Sum/2, Mux1/3
  Demux/2 -> Sum1/2, Mux1/2
  Demux/1 -> Mux1/1, Sum2/2

== system tongbukongzhi2/Subsystem1/Subsystem2/fuzzypid4/Subsystem ==
  In1 : Inport
  In2 : Inport  Port=2
  Add : Sum  Inputs=+++
  Demux : Demux  Outputs=3
  Derivative : Derivative
  Fuzzy Logic Controller : fuzblock/Fuzzy Logic  Controller  fis=fuzzy1
  Gain : Gain  Gain=12.9851074749726
  Gain1 : Gain  Gain=3.96505413373294
  Gain2 : Gain  Gain=0.756963167778154
  Integrator : Integrator
  Mux : Mux  Inputs=2
  Mux1 : Mux  Inputs=3
  Scope : Scope
      settings: YMin=-0.2  YMax=0.05
  Sum : Sum  Inputs=|++
  Sum1 : Sum  Inputs=|++
  Sum2 : Sum  Inputs=|++
  Zero-Order Hold : ZeroOrderHold  SampleTime=0.1
  Zero-Order Hold1 : ZeroOrderHold  SampleTime=0.1
  Out1 : Outport
  wires:
  In1/1 -> Gain/1, Gain2/1, Gain1/1, Mux/1
  Derivative/1 -> Add/3
  Integrator/1 -> Add/2
  Add/1 -> Out1/1
  In2/1 -> Mux/2
  Gain/1 -> Sum2/1
  Sum2/1 -> Add/1
  Gain1/1 -> Sum1/1
  Sum1/1 -> Integrator/1
  Gain2/1 -> Sum/1
  Sum/1 -> Derivative/1
  Mux/1 -> Zero-Order Hold/1
  Fuzzy Logic Controller/1 -> Zero-Order Hold1/1
  Zero-Order Hold/1 -> Fuzzy Logic Controller/1
  Zero-Order Hold1/1 -> Demux/1
  Mux1/1 -> Scope/1
  Demux/3 -> Sum/2, Mux1/3
  Demux/2 -> Sum1/2, Mux1/2
  Demux/1 -> Mux1/1, Sum2/2

== system tongbukongzhi2/Subsystem1/Subsystem2/fuzzypid5/Subsystem ==
  In1 : Inport
  In2 : Inport  Port=2
  Add : Sum  Inputs=+++
  Demux : Demux  Outputs=3
  Derivative : Derivative
  Fuzzy Logic Controller : fuzblock/Fuzzy Logic  Controller  fis=fuzzy1
  Gain : Gain  Gain=12.9851074749726
  Gain1 : Gain  Gain=3.96505413373294
  Gain2 : Gain  Gain=0.756963167778154
  Integrator : Integrator
  Mux : Mux  Inputs=2
  Mux1 : Mux  Inputs=3
  Scope : Scope
      settings: YMin=-0.2  YMax=0.05
  Sum : Sum  Inputs=|++
  Sum1 : Sum  Inputs=|++
  Sum2 : Sum  Inputs=|++
  Zero-Order Hold : ZeroOrderHold  SampleTime=0.1
  Zero-Order Hold1 : ZeroOrderHold  SampleTime=0.1
  Out1 : Outport
  wires:
  In1/1 -> Gain/1, Gain2/1, Gain1/1, Mux/1
  Derivative/1 -> Add/3
  Integrator/1 -> Add/2
  Add/1 -> Out1/1
  In2/1 -> Mux/2
  Gain/1 -> Sum2/1
  Sum2/1 -> Add/1
  Gain1/1 -> Sum1/1
  Sum1/1 -> Integrator/1
  Gain2/1 -> Sum/1
  Sum/1 -> Derivative/1
  Mux/1 -> Zero-Order Hold/1
  Fuzzy Logic Controller/1 -> Zero-Order Hold1/1
  Zero-Order Hold/1 -> Fuzzy Logic Controller/1
  Zero-Order Hold1/1 -> Demux/1
  Mux1/1 -> Scope/1
  Demux/3 -> Sum/2, Mux1/3
  Demux/2 -> Sum1/2, Mux1/2
  Demux/1 -> Mux1/1, Sum2/2

== system tongbukongzhi2/Subsystem1/Subsystem2/fuzzypid6/Subsystem ==
  In1 : Inport
  In2 : Inport  Port=2
  Add : Sum  Inputs=+++
  Demux : Demux  Outputs=3
  Derivative : Derivative
  Fuzzy Logic Controller : fuzblock/Fuzzy Logic  Controller  fis=fuzzy1
  Gain : Gain  Gain=12.9851074749726
  Gain1 : Gain  Gain=3.96505413373294
  Gain2 : Gain  Gain=0.756963167778154
  Integrator : Integrator
  Mux : Mux  Inputs=2
  Mux1 : Mux  Inputs=3
  Scope : Scope
      settings: YMin=-0.2  YMax=0.05
  Sum : Sum  Inputs=|++
  Sum1 : Sum  Inputs=|++
  Sum2 : Sum  Inputs=|++
  Zero-Order Hold : ZeroOrderHold  SampleTime=0.1
  Zero-Order Hold1 : ZeroOrderHold  SampleTime=0.1
  Out1 : Outport
  wires:
  In1/1 -> Gain/1, Gain2/1, Gain1/1, Mux/1
  Derivative/1 -> Add/3
  Integrator/1 -> Add/2
  Add/1 -> Out1/1
  In2/1 -> Mux/2
  Gain/1 -> Sum2/1
  Sum2/1 -> Add/1
  Gain1/1 -> Sum1/1
  Sum1/1 -> Integrator/1
  Gain2/1 -> Sum/1
  Sum/1 -> Derivative/1
  Mux/1 -> Zero-Order Hold/1
  Fuzzy Logic Controller/1 -> Zero-Order Hold1/1
  Zero-Order Hold/1 -> Fuzzy Logic Controller/1
  Zero-Order Hold1/1 -> Demux/1
  Mux1/1 -> Scope/1
  Demux/3 -> Sum/2, Mux1/3
  Demux/2 -> Sum1/2, Mux1/2
  Demux/1 -> Mux1/1, Sum2/2

== system tongbukongzhi2/Subsystem1/Subsystem3/fuzzypid4/Subsystem ==
  In1 : Inport
  In2 : Inport  Port=2
  Add : Sum  Inputs=+++
  Demux : Demux  Outputs=3
  Derivative : Derivative
  Fuzzy Logic Controller : fuzblock/Fuzzy Logic  Controller  fis=fuzzy1
  Gain : Gain  Gain=12.9851074749726
  Gain1 : Gain  Gain=3.96505413373294
  Gain2 : Gain  Gain=0.756963167778154
  Integrator : Integrator
  Mux : Mux  Inputs=2
  Mux1 : Mux  Inputs=3
  Scope : Scope
      settings: YMin=-0.2  YMax=0.05
  Sum : Sum  Inputs=|++
  Sum1 : Sum  Inputs=|++
  Sum2 : Sum  Inputs=|++
  Zero-Order Hold : ZeroOrderHold  SampleTime=0.1
  Zero-Order Hold1 : ZeroOrderHold  SampleTime=0.1
  Out1 : Outport
  wires:
  In1/1 -> Gain/1, Gain2/1, Gain1/1, Mux/1
  Derivative/1 -> Add/3
  Integrator/1 -> Add/2
  Add/1 -> Out1/1
  In2/1 -> Mux/2
  Gain/1 -> Sum2/1
  Sum2/1 -> Add/1
  Gain1/1 -> Sum1/1
  Sum1/1 -> Integrator/1
  Gain2/1 -> Sum/1
  Sum/1 -> Derivative/1
  Mux/1 -> Zero-Order Hold/1
  Fuzzy Logic Controller/1 -> Zero-Order Hold1/1
  Zero-Order Hold/1 -> Fuzzy Logic Controller/1
  Zero-Order Hold1/1 -> Demux/1
  Mux1/1 -> Scope/1
  Demux/3 -> Sum/2, Mux1/3
  Demux/2 -> Sum1/2, Mux1/2
  Demux/1 -> Mux1/1, Sum2/2

== system tongbukongzhi2/Subsystem1/Subsystem3/fuzzypid5/Subsystem ==
  In1 : Inport
  In2 : Inport  Port=2
  Add : Sum  Inputs=+++
  Demux : Demux  Outputs=3
  Derivative : Derivative
  Fuzzy Logic Controller : fuzblock/Fuzzy Logic  Controller  fis=fuzzy1
  Gain : Gain  Gain=12.9851074749726
  Gain1 : Gain  Gain=3.96505413373294
  Gain2 : Gain  Gain=0.756963167778154
  Integrator : Integrator
  Mux : Mux  Inputs=2
  Mux1 : Mux  Inputs=3
  Scope : Scope
      settings: YMin=-0.2  YMax=0.05
  Sum : Sum  Inputs=|++
  Sum1 : Sum  Inputs=|++
  Sum2 : Sum  Inputs=|++
  Zero-Order Hold : ZeroOrderHold  SampleTime=0.1
  Zero-Order Hold1 : ZeroOrderHold  SampleTime=0.1
  Out1 : Outport
  wires:
  In1/1 -> Gain/1, Gain2/1, Gain1/1, Mux/1
  Derivative/1 -> Add/3
  Integrator/1 -> Add/2
  Add/1 -> Out1/1
  In2/1 -> Mux/2
  Gain/1 -> Sum2/1
  Sum2/1 -> Add/1
  Gain1/1 -> Sum1/1
  Sum1/1 -> Integrator/1
  Gain2/1 -> Sum/1
  Sum/1 -> Derivative/1
  Mux/1 -> Zero-Order Hold/1
  Fuzzy Logic Controller/1 -> Zero-Order Hold1/1
  Zero-Order Hold/1 -> Fuzzy Logic Controller/1
  Zero-Order Hold1/1 -> Demux/1
  Mux1/1 -> Scope/1
  Demux/3 -> Sum/2, Mux1/3
  Demux/2 -> Sum1/2, Mux1/2
  Demux/1 -> Mux1/1, Sum2/2

== system tongbukongzhi2/Subsystem1/Subsystem3/fuzzypid6/Subsystem ==
  In1 : Inport
  In2 : Inport  Port=2
  Add : Sum  Inputs=+++
  Demux : Demux  Outputs=3
  Derivative : Derivative
  Fuzzy Logic Controller : fuzblock/Fuzzy Logic  Controller  fis=fuzzy1
  Gain : Gain  Gain=12.9851074749726
  Gain1 : Gain  Gain=3.96505413373294
  Gain2 : Gain  Gain=0.756963167778154
  Integrator : Integrator
  Mux : Mux  Inputs=2
  Mux1 : Mux  Inputs=3
  Scope : Scope
      settings: YMin=-0.2  YMax=0.05
  Sum : Sum  Inputs=|++
  Sum1 : Sum  Inputs=|++
  Sum2 : Sum  Inputs=|++
  Zero-Order Hold : ZeroOrderHold  SampleTime=0.1
  Zero-Order Hold1 : ZeroOrderHold  SampleTime=0.1
  Out1 : Outport
  wires:
  In1/1 -> Gain/1, Gain2/1, Gain1/1, Mux/1
  Derivative/1 -> Add/3
  Integrator/1 -> Add/2
  Add/1 -> Out1/1
  In2/1 -> Mux/2
  Gain/1 -> Sum2/1
  Sum2/1 -> Add/1
  Gain1/1 -> Sum1/1
  Sum1/1 -> Integrator/1
  Gain2/1 -> Sum/1
  Sum/1 -> Derivative/1
  Mux/1 -> Zero-Order Hold/1
  Fuzzy Logic Controller/1 -> Zero-Order Hold1/1
  Zero-Order Hold/1 -> Fuzzy Logic Controller/1
  Zero-Order Hold1/1 -> Demux/1
  Mux1/1 -> Scope/1
  Demux/3 -> Sum/2, Mux1/3
  Demux/2 -> Sum1/2, Mux1/2
  Demux/1 -> Mux1/1, Sum2/2

== system tongbukongzhi2/Subsystem1/Subsystem8/fuzzypid2/Subsystem ==
  In1 : Inport
  In2 : Inport  Port=2
  Add : Sum  Inputs=+++
  Demux : Demux  Outputs=3
  Derivative : Derivative
  Fuzzy Logic Controller : fuzblock/Fuzzy Logic  Controller  fis=fuzzy1
  Gain : Gain  Gain=0.341898282831464
  Gain1 : Gain  Gain=4.22711463410027
  Gain2 : Gain  Gain=-0.0039506922991482
  Integrator : Integrator
  Mux : Mux  Inputs=2
  Mux1 : Mux  Inputs=3
  Scope : Scope
      settings: YMin=-0.2  YMax=0.05
  Sum : Sum  Inputs=|++
  Sum1 : Sum  Inputs=|++
  Sum2 : Sum  Inputs=|++
  Zero-Order Hold : ZeroOrderHold  SampleTime=0.1
  Zero-Order Hold1 : ZeroOrderHold  SampleTime=0.1
  Out1 : Outport
  wires:
  In1/1 -> Gain/1, Gain2/1, Gain1/1, Mux/1
  Derivative/1 -> Add/3
  Integrator/1 -> Add/2
  Add/1 -> Out1/1
  In2/1 -> Mux/2
  Gain/1 -> Sum2/1
  Sum2/1 -> Add/1
  Gain1/1 -> Sum1/1
  Sum1/1 -> Integrator/1
  Gain2/1 -> Sum/1
  Sum/1 -> Derivative/1
  Mux/1 -> Zero-Order Hold/1
  Fuzzy Logic Controller/1 -> Zero-Order Hold1/1
  Zero-Order Hold/1 -> Fuzzy Logic Controller/1
  Zero-Order Hold1/1 -> Demux/1
  Mux1/1 -> Scope/1
  Demux/3 -> Sum/2, Mux1/3
  Demux/2 -> Sum1/2, Mux1/2
  Demux/1 -> Mux1/1, Sum2/2
